simulink model "IRIS_rads"  (Simulink 8.5)
settings: Solver=ode45  StartTime=0.0  StopTime=100  MinStep=0.0001  RelTol=1e-3
undefined symbols (not defined in the file or in its folder): quad
settings Model: Creator=evgenov  LastModifiedBy=Alexey
settings DebuggingCC: SolverPrmCheckMsg=warning  FcnCallInpInsideContextMsg=EnableAllAsWarning
settings ConfigurationSet: Description=SimMechanics 2G

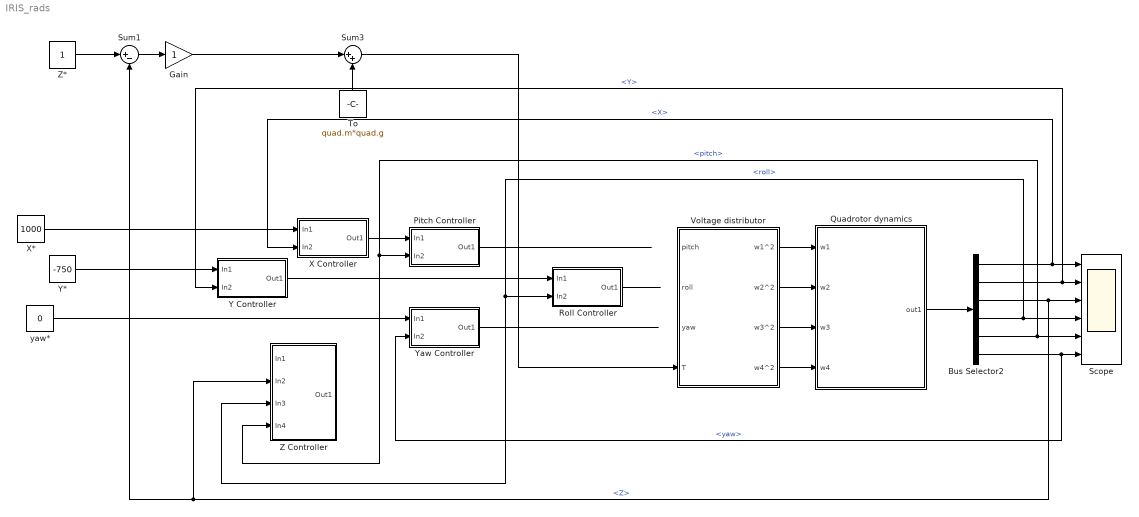
== system IRIS_rads ==
  Bus Selector2 : BusSelector  OutputSignals=X,Y,Z,roll,pitch,yaw
  Gain : Gain
  Pitch Controller : Subsystem
  Quadrotor dynamics : Subsystem
  Roll Controller : Subsystem
  Scope : Scope  NumInputPorts=6
      settings: TimeRange=100  YMin=21~-33~19.6~-0.03~-0.04~-5e-05  YMax=26~-25~19.775~0.04~0.05~0.0003  SaveName=ScopeData2
  Sum1 : Sum  Inputs=|+-
  Sum3 : Sum  Inputs=|++
  To : Constant  Value=quad.m*quad.g
  Voltage distributor : Subsystem
  X Controller : Subsystem
  X* : Constant  Value=1000
  Y Controller : Subsystem
  Y* : Constant  Value=-750
  Yaw Controller : Subsystem
  Z Controller : Subsystem
  Z* : Constant
  yaw* : Constant  Value=0
  wires:
  Quadrotor dynamics/1(out1) -> Bus Selector2/1
  Bus Selector2/1 -> X Controller/2(In2), Scope/1  "<X>"
  Bus Selector2/2 -> Y Controller/2(In2), Scope/2  "<Y>"
  Bus Selector2/3 -> Sum1/2, Z Controller/2(In2), Scope/3  "<Z>"
  Bus Selector2/4 -> Roll Controller/2(In2), Z Controller/3(In3), Scope/4  "<roll>"
  Bus Selector2/6 -> Yaw Controller/2(In2), Scope/6  "<yaw>"
  Voltage distributor/1("w1^2 ") -> Quadrotor dynamics/1(w1)
  Voltage distributor/2("w2^2 ") -> Quadrotor dynamics/2(w2)
  Voltage distributor/3("w3^2 ") -> Quadrotor dynamics/3(w3)
  Voltage distributor/4("w4^2 ") -> Quadrotor dynamics/4(w4)
  Bus Selector2/5 -> Z Controller/4(In4), Pitch Controller/2(In2), Scope/5  "<pitch>"
  Sum3/1 -> Voltage distributor/4(T)
  yaw*/1 -> Yaw Controller/1(In1)
  Yaw Controller/1(Out1) -> ?
  Roll Controller/1(Out1) -> ?
  Pitch Controller/1(Out1) -> ?
  X Controller/1(Out1) -> Pitch Controller/1(In1)
  Y Controller/1(Out1) -> Roll Controller/1(In1)
  X*/1 -> X Controller/1(In1)
  Y*/1 -> Y Controller/1(In1)
  To/1 -> Sum3/2
  Z*/1 -> Sum1/1
  Gain/1 -> Sum3/1
  Sum1/1 -> Gain/1

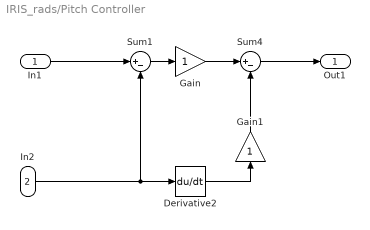
== system IRIS_rads/Pitch Controller ==
  In1 : Inport
  In2 : Inport  Port=2
  Derivative2 : Derivative
  Gain : Gain
  Gain1 : Gain
  Sum1 : Sum  Inputs=|+-
  Sum4 : Sum  Inputs=|+-
  Out1 : Outport
  wires:
  In1/1 -> Sum1/1
  In2/1 -> Derivative2/1, Sum1/2
  Sum1/1 -> Gain/1
  Gain/1 -> Sum4/1
  Derivative2/1 -> Gain1/1
  Gain1/1 -> Sum4/2
  Sum4/1 -> Out1/1

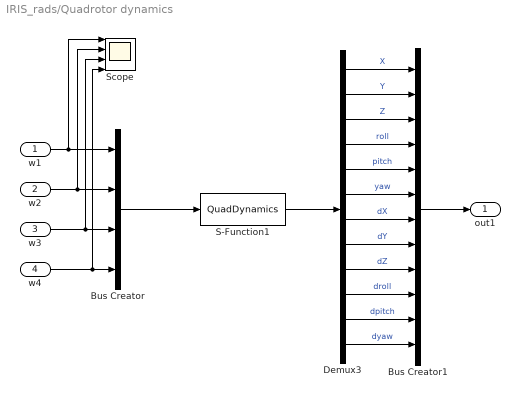
== system IRIS_rads/Quadrotor dynamics ==
  w1 : Inport
  w2 : Inport  Port=2
  w3 : Inport  Port=3
  w4 : Inport  Port=4
  Bus Creator : BusCreator
  Bus Creator1 : BusCreator  Inputs=12
  Demux3 : Demux  Outputs=12
  S-Function1 : S-Function  FunctionName=QuadDynamics  Parameters=quad
  Scope : Scope  NumInputPorts=4
      settings: YMin=-5~-5~-5~-5  YMax=5~5~5~5
  out1 : Outport
  wires:
  w1/1 -> Scope/1, Bus Creator/1
  w2/1 -> Scope/2, Bus Creator/2
  w3/1 -> Scope/3, Bus Creator/3
  w4/1 -> Scope/4, Bus Creator/4
  Bus Creator1/1 -> out1/1
  Bus Creator/1 -> S-Function1/1
  Demux3/1 -> Bus Creator1/1  "X"
  Demux3/2 -> Bus Creator1/2  "Y"
  Demux3/3 -> Bus Creator1/3  "Z"
  Demux3/4 -> Bus Creator1/4  "roll"
  Demux3/5 -> Bus Creator1/5  "pitch"
  Demux3/6 -> Bus Creator1/6  "yaw"
  Demux3/7 -> Bus Creator1/7  "dX"
  Demux3/8 -> Bus Creator1/8  "dY"
  Demux3/9 -> Bus Creator1/9  "dZ"
  Demux3/10 -> Bus Creator1/10  "droll"
  Demux3/11 -> Bus Creator1/11  "dpitch"
  Demux3/12 -> Bus Creator1/12  "dyaw"
  S-Function1/1 -> Demux3/1

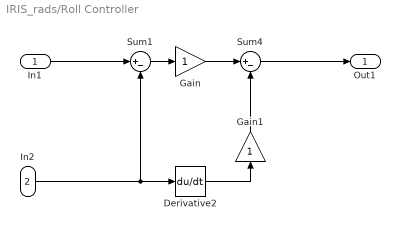
== system IRIS_rads/Roll Controller ==
  In1 : Inport
  In2 : Inport  Port=2
  Derivative2 : Derivative
  Gain : Gain
  Gain1 : Gain
  Sum1 : Sum  Inputs=|+-
  Sum4 : Sum  Inputs=|+-
  Out1 : Outport
  wires:
  In1/1 -> Sum1/1
  In2/1 -> Derivative2/1, Sum1/2
  Sum1/1 -> Gain/1
  Sum4/1 -> Out1/1
  Gain/1 -> Sum4/1
  Derivative2/1 -> Gain1/1
  Gain1/1 -> Sum4/2

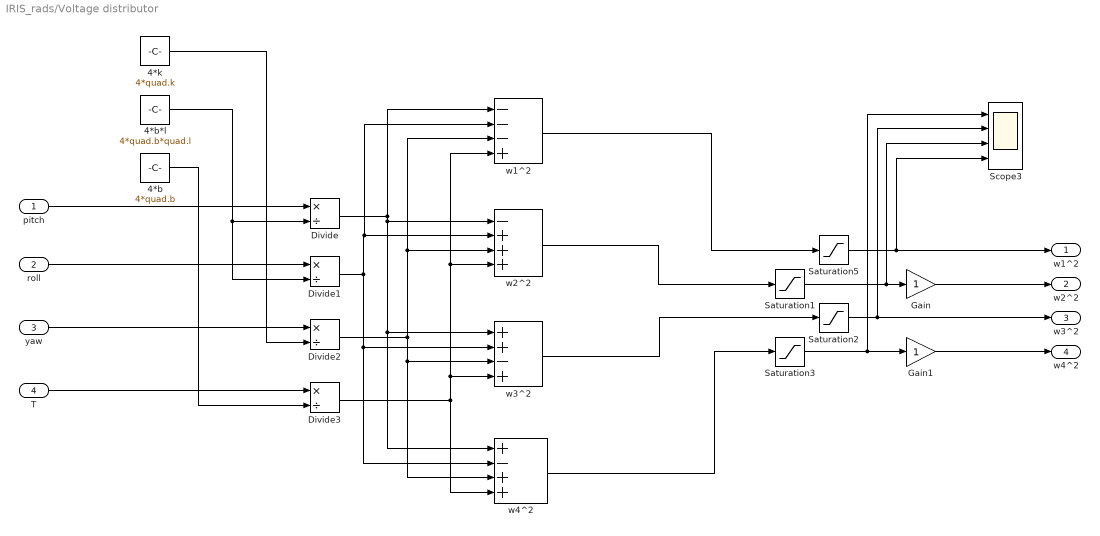
== system IRIS_rads/Voltage distributor ==
  pitch : Inport
  roll : Inport  Port=2
  yaw : Inport  Port=3
  T : Inport  Port=4
  4*b : Constant  Value=4*quad.b
  4*b*l : Constant  Value=4*quad.b*quad.l
  4*k : Constant  Value=4*quad.k
  Divide{,1..3} (4 alike) : Product  Inputs=*/
  Gain : Gain
  Gain1 : Gain
  Saturation{1..3,5} (4 alike) : Saturate  UpperLimit=976144  LowerLimit=244036  ZeroCross=off
  Scope3 : Scope  NumInputPorts=4
      settings: YMin=-5~-5~-5~-5  YMax=5~5~5~5  SaveName=ScopeData7
  w1^2 : Sum  Inputs=---+
  w2^2 : Sum  Inputs=-+++
  w3^2 : Sum  Inputs=++-+
  w4^2 : Sum  Inputs=+-++
  "w1^2 " : Outport
  "w2^2 " : Outport  Port=2
  "w3^2 " : Outport  Port=3
  "w4^2 " : Outport  Port=4
  wires:
  4*k/1 -> Divide2/2
  Divide1/1 -> w3^2/2, w4^2/2, w1^2/2, w2^2/2
  Divide2/1 -> w4^2/3, w3^2/3, w2^2/3, w1^2/3
  Divide/1 -> w2^2/1, w4^2/1, w3^2/1, w1^2/1
  4*b/1 -> Divide3/2
  yaw/1 -> Divide2/1
  4*b*l/1 -> Divide/2, Divide1/2
  roll/1 -> Divide1/1
  pitch/1 -> Divide/1
  Divide3/1 -> w4^2/4, w3^2/4, w2^2/4, w1^2/4
  Gain/1 -> "w2^2 "/1
  Gain1/1 -> "w4^2 "/1
  Saturation5/1 -> "w1^2 "/1, Scope3/4
  Saturation1/1 -> Gain/1, Scope3/3
  Saturation2/1 -> "w3^2 "/1, Scope3/2
  Saturation3/1 -> Gain1/1, Scope3/1
  w1^2/1 -> Saturation5/1
  w2^2/1 -> Saturation1/1
  w3^2/1 -> Saturation2/1
  w4^2/1 -> Saturation3/1
  T/1 -> Divide3/1

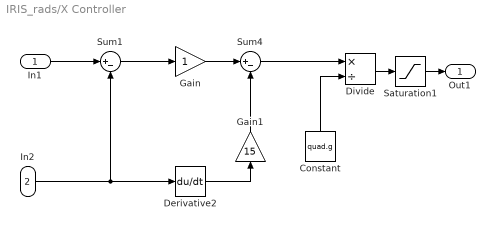
== system IRIS_rads/X Controller ==
  In1 : Inport
  In2 : Inport  Port=2
  Constant : Constant  Value=quad.g
  Derivative2 : Derivative
  Divide : Product  Inputs=*/
  Gain : Gain
  Gain1 : Gain  Gain=15
  Saturation1 : Saturate  UpperLimit=0.1  LowerLimit=-0.1  ZeroCross=off
  Sum1 : Sum  Inputs=|+-
  Sum4 : Sum  Inputs=|+-
  Out1 : Outport
  wires:
  In2/1 -> Sum1/2, Derivative2/1
  Gain/1 -> Sum4/1
  Derivative2/1 -> Gain1/1
  Gain1/1 -> Sum4/2
  Sum4/1 -> Divide/1
  Constant/1 -> Divide/2
  Divide/1 -> Saturation1/1
  Saturation1/1 -> Out1/1
  In1/1 -> Sum1/1
  Sum1/1 -> Gain/1

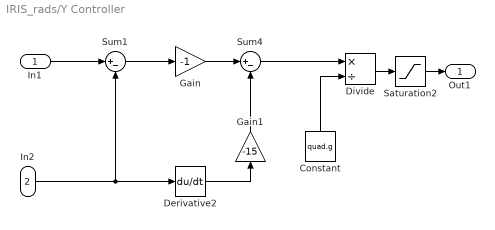
== system IRIS_rads/Y Controller ==
  In1 : Inport
  In2 : Inport  Port=2
  Constant : Constant  Value=quad.g
  Derivative2 : Derivative
  Divide : Product  Inputs=*/
  Gain : Gain  Gain=-1
  Gain1 : Gain  Gain=-15
  Saturation2 : Saturate  UpperLimit=0.1  LowerLimit=-0.1  ZeroCross=off
  Sum1 : Sum  Inputs=|+-
  Sum4 : Sum  Inputs=|+-
  Out1 : Outport
  wires:
  In2/1 -> Sum1/2, Derivative2/1
  Gain/1 -> Sum4/1
  Derivative2/1 -> Gain1/1
  Gain1/1 -> Sum4/2
  Sum4/1 -> Divide/1
  Constant/1 -> Divide/2
  Divide/1 -> Saturation2/1
  Saturation2/1 -> Out1/1
  In1/1 -> Sum1/1
  Sum1/1 -> Gain/1

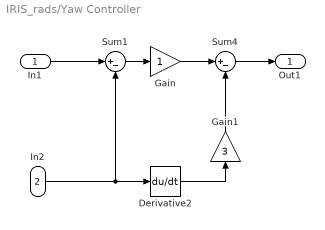
== system IRIS_rads/Yaw Controller ==
  In1 : Inport
  In2 : Inport  Port=2
  Derivative2 : Derivative
  Gain : Gain
  Gain1 : Gain  Gain=3
  Sum1 : Sum  Inputs=|+-
  Sum4 : Sum  Inputs=|+-
  Out1 : Outport
  wires:
  In1/1 -> Sum1/1
  In2/1 -> Derivative2/1, Sum1/2
  Sum1/1 -> Gain/1
  Sum4/1 -> Out1/1
  Gain/1 -> Sum4/1
  Derivative2/1 -> Gain1/1
  Gain1/1 -> Sum4/2

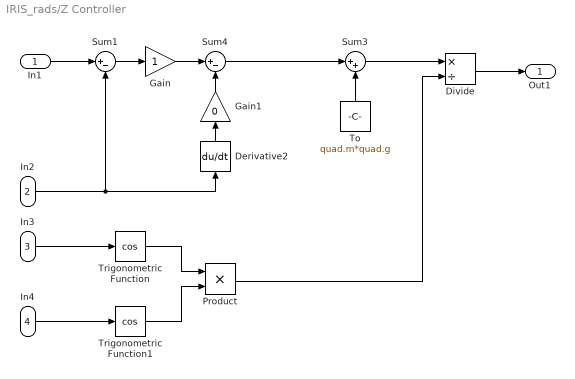
== system IRIS_rads/Z Controller ==
  In1 : Inport
  In2 : Inport  Port=2
  In3 : Inport  Port=3
  In4 : Inport  Port=4
  Derivative2 : Derivative
  Divide : Product  Inputs=*/
  Gain : Gain
  Gain1 : Gain  Gain=0
  Product : Product
  Sum1 : Sum  Inputs=|+-
  Sum3 : Sum  Inputs=|++
  Sum4 : Sum  Inputs=|+-
  To : Constant  Value=quad.m*quad.g
  Trigonometric Function : Trigonometry  Operator=cos
  Trigonometric Function1 : Trigonometry  Operator=cos
  Out1 : Outport
  wires:
  In4/1 -> Trigonometric Function1/1
  In3/1 -> Trigonometric Function/1
  Trigonometric Function/1 -> Product/1
  Trigonometric Function1/1 -> Product/2
  Product/1 -> Divide/2
  To/1 -> Sum3/2
  Sum3/1 -> Divide/1
  Divide/1 -> Out1/1
  In1/1 -> Sum1/1
  Gain/1 -> Sum4/1
  Derivative2/1 -> Gain1/1
  Gain1/1 -> Sum4/2
  Sum4/1 -> Sum3/1
  In2/1 -> Sum1/2, Derivative2/1
  Sum1/1 -> Gain/1
